simulink model "SemSisClass3Sim"  (R2022b)
settings: Solver=ode4  StartTime=0.0  StopTime=5  FixedStep=0.02  RelTol=1e-3
values from neighbouring files (symbols this model uses):
  g = 9.81    [SemSisClass3.m]
  l1 = 0.3    [SemSisClass3.m]
  l2 = 0.25    [SemSisClass3.m]
  m1 = 0.2    [SemSisClass3.m]
  m2 = 0.1    [SemSisClass3.m]
settings Model: Creator=mluser  LastModifiedBy=ferch

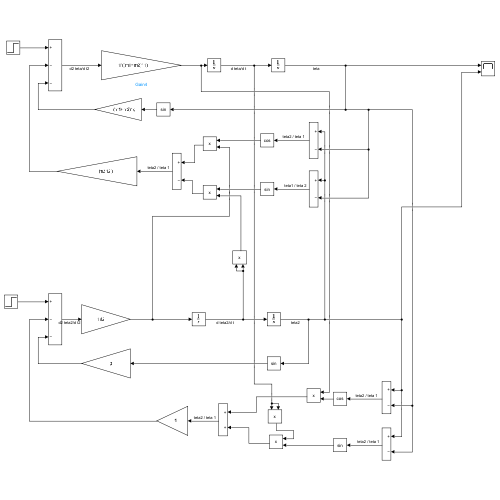
[thumbnail: Simulink's stored preview of the top-level diagram]
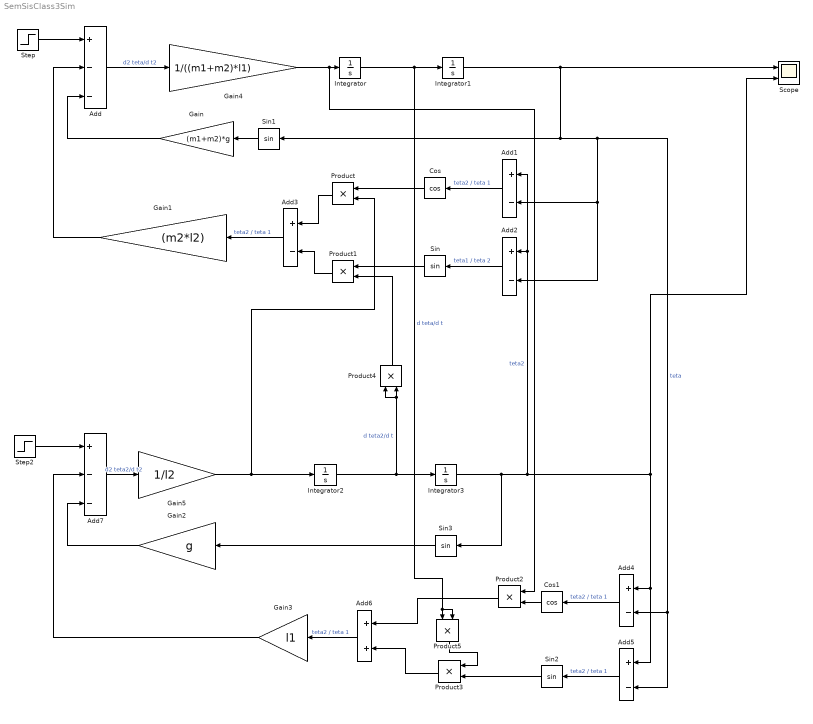
== system SemSisClass3Sim ==
  Add : Sum  Inputs=+--
  Add{1..5} (5 alike) : Sum  Inputs=+-
  Add6 : Sum
  Add7 : Sum  Inputs=+--
  Cos : Trigonometry  Operator=cos
  Cos1 : Trigonometry  Operator=cos
  Gain : Gain  Gain=(m1+m2)*g
  Gain1 : Gain  Gain=(m2*l2)
  Gain2 : Gain  Gain=g
  Gain3 : Gain  Gain=l1
  Gain4 : Gain  Gain=1/((m1+m2)*l1)
  Gain5 : Gain  Gain=1/l2
  Integrator : Integrator
  Integrator1 : Integrator
  Integrator2 : Integrator
  Integrator3 : Integrator  InitialCondition=(35*pi)/180
  Product{,1..5} (6 alike) : Product
  Scope : Scope  NumInputPorts=2
  Sin{,1..3} (4 alike) : Trigonometry
  Step : Step  After=0  SampleTime=0
  Step2 : Step  After=0  SampleTime=0
  wires:
  Add/1 -> Gain4/1  "d2 teta/d t2"
  Integrator/1 -> Product5/2, Product5/1, Integrator1/1  "d teta/d t"
  Integrator1/1 -> Scope/1, Add1/2, Add2/2, Add5/2, Add4/2, Sin1/1  "teta"
  Add1/1 -> Cos/1  "teta2 / teta 1"
  Add2/1 -> Sin/1  "teta1 / teta 2"
  Product/1 -> Add3/1
  Add3/1 -> Gain1/1  "teta2 / teta 1"
  Gain1/1 -> Add/2
  Cos/1 -> Product/1
  Integrator2/1 -> Integrator3/1, Product4/1, Product4/2  "d teta2/d t"
  Add7/1 -> Gain5/1  "d2 teta2/d t2"
  Gain3/1 -> Add7/2
  Product4/1 -> Product1/2
  Gain2/1 -> Add7/3
  Add4/1 -> Cos1/1  "teta2 / teta 1"
  Add5/1 -> Sin2/1  "teta2 / teta 1"
  Product5/1 -> Product3/1
  Product2/1 -> Add6/1
  Product3/1 -> Add6/2
  Add6/1 -> Gain3/1  "teta2 / teta 1"
  Sin/1 -> Product1/1
  Sin1/1 -> Gain/1
  Gain4/1 -> Product2/1, Integrator/1
  Sin2/1 -> Product3/2
  Sin3/1 -> Gain2/1
  Gain5/1 -> Integrator2/1, Product/2
  Integrator3/1 -> Scope/2, Add5/1, Add4/1, Add2/1, Add1/1, Sin3/1  "teta2"
  Cos1/1 -> Product2/2
  Product1/1 -> Add3/2
  Gain/1 -> Add/3
  Step/1 -> Add/1
  Step2/1 -> Add7/1
